simulink model "CTRL_SPECCTRL_FF_STEER_test"  (R2024b)
settings: Solver=VariableStepAuto  StartTime=0.0  StopTime=10.0  RelTol=1e-3
libraries: CTRL_SPECCTRL_FF_STEER x1
settings Model: Creator=blatak  LastModifiedBy=blatak

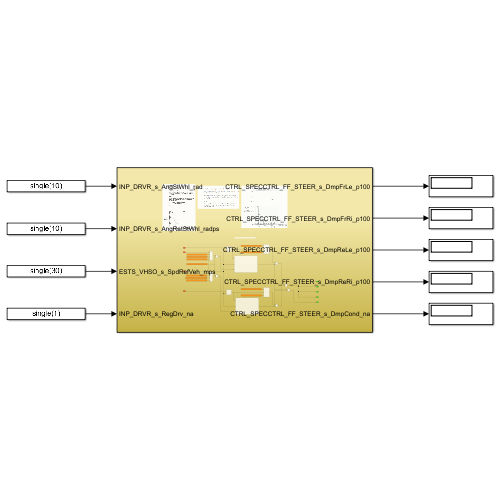
[thumbnail: Simulink's stored preview of the top-level diagram]
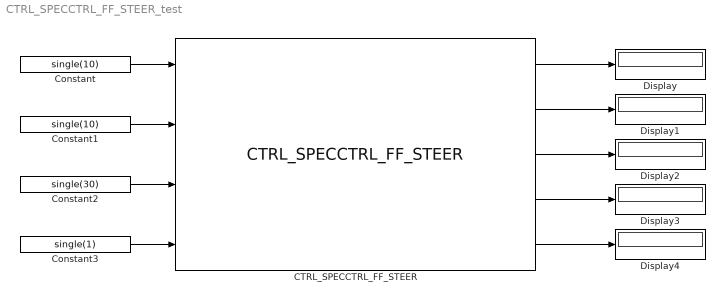
== system CTRL_SPECCTRL_FF_STEER_test ==
  CTRL_SPECCTRL_FF_STEER : CTRL_SPECCTRL_FF_STEER/CTRL_SPECCTRL_FF_STEER  SystemSampleTime=-1  VariantActivationTime=update diagram  AllowFlexibleInterface=on  Latency=0  AutoFrameSizeCalculation=off
  Constant : Constant  Value=single(10)
  Constant1 : Constant  Value=single(10)
  Constant2 : Constant  Value=single(30)
  Constant3 : Constant  Value=single(1)
  Display{,1..4} (5 alike) : Display
  wires:
  CTRL_SPECCTRL_FF_STEER/1 -> Display/1
  CTRL_SPECCTRL_FF_STEER/2 -> Display1/1
  CTRL_SPECCTRL_FF_STEER/3 -> Display2/1
  CTRL_SPECCTRL_FF_STEER/4 -> Display3/1
  Constant/1 -> CTRL_SPECCTRL_FF_STEER/1
  Constant1/1 -> CTRL_SPECCTRL_FF_STEER/2
  Constant2/1 -> CTRL_SPECCTRL_FF_STEER/3
  Constant3/1 -> CTRL_SPECCTRL_FF_STEER/4
  CTRL_SPECCTRL_FF_STEER/5 -> Display4/1
